simulink model "delayobserver_sim"  (R2016a)
settings: Solver=VariableStepAuto  StartTime=0.0  StopTime=10.0  RelTol=1e-3
settings Model: Creator=zhanghankui  LastModifiedBy=zhanghankui

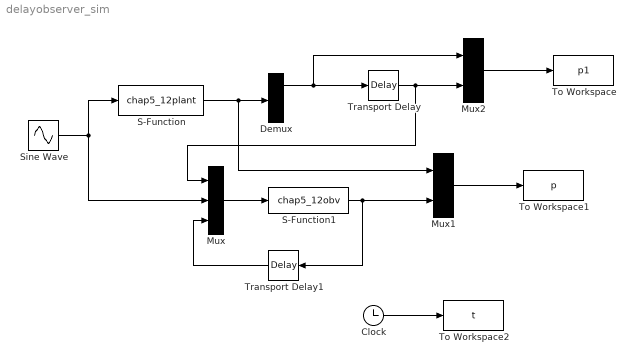
== system delayobserver_sim ==
  Clock : Clock
  Demux : Demux  Outputs=2
  Mux : Mux  Inputs=3
  Mux1 : Mux  Inputs=2
  Mux2 : Mux  Inputs=2
  S-Function : S-Function  FunctionName=chap5_12plant  SFunctionDeploymentMode=off  EnableBusSupport=off
  S-Function1 : S-Function  FunctionName=chap5_12obv  SFunctionDeploymentMode=off  EnableBusSupport=off
  Sine Wave : Sin  SampleTime=0
  To Workspace : ToWorkspace  VariableName=p1  SampleTime=-1
  To Workspace1 : ToWorkspace  VariableName=p  SampleTime=-1
  To Workspace2 : ToWorkspace  VariableName=t  SampleTime=-1
  Transport Delay : TransportDelay  DelayTime=3.0
  Transport Delay1 : TransportDelay  DelayTime=3.0
  wires:
  Sine Wave/1 -> Mux/2, S-Function/1
  Mux/1 -> S-Function1/1
  S-Function/1 -> Mux1/1, Demux/1
  Demux/1 -> Mux2/1, Transport Delay/1
  S-Function1/1 -> Mux1/2, Transport Delay1/1
  Transport Delay1/1 -> Mux/3
  Transport Delay/1 -> Mux2/2, Mux/1
  Mux2/1 -> To Workspace/1
  Mux1/1 -> To Workspace1/1
  Clock/1 -> To Workspace2/1
